simulink model "sampleModel1855"  (R2023a)
settings: Solver=VariableStepAuto  StartTime=0.0  StopTime=10.0  RelTol=1e-3
libraries: hdlsllib x4, simulink x1
settings Model: Creator=user1  LastModifiedBy=user1

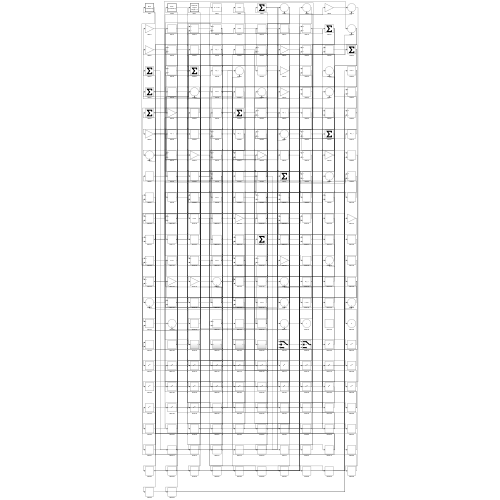
[thumbnail: Simulink's stored preview of the top-level diagram]
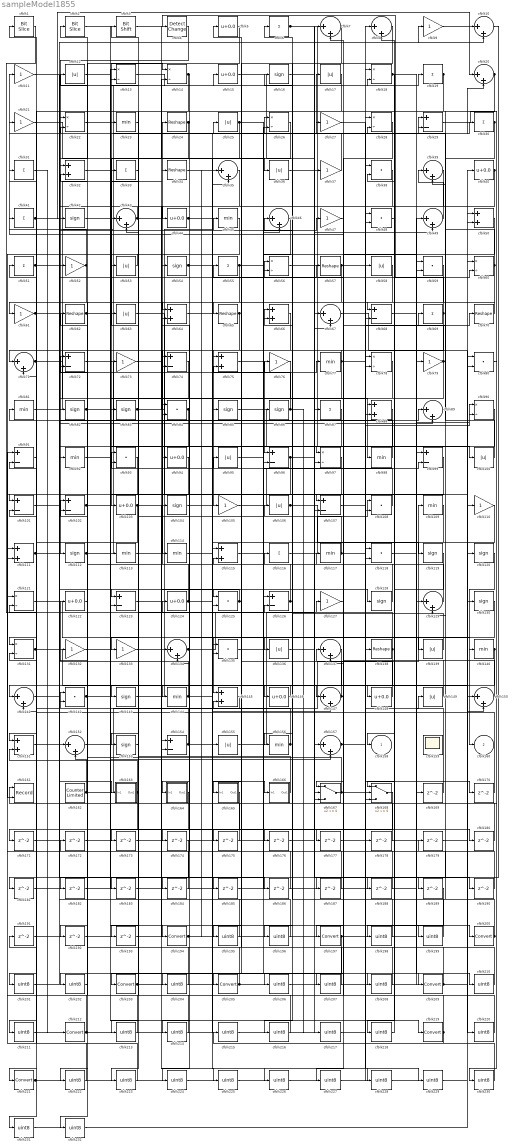
== system sampleModel1855 ==
  cfblk1 : hdlsllib/Logic and Bit Operations/Bit Slice  lidx=7  ridx=0
  cfblk{7..8,10,20,35,39,43,46,49,67,71,89,129,134,137,141,147,150,152,157} (20 alike) : Sum  Inputs=|++
  cfblk{12,17,25,36,53,58,63,95,100,106,136,139,149,155} (14 alike) : Abs  SaturateOnIntegerOverflow=off
  cfblk{29,68,72,74,91,96,99,101..102,107,123,126,154} (13 alike) : Sum  Inputs=+-
  cfblk{5,15,40,44,94,103,122,124,146,148} (10 alike) : Bias  Bias=0.0  SaturateOnIntegerOverflow=off
  cfblk{16,42,54,82..83,85..86,104,112,119..120,128,130,143,153} (15 alike) : Signum
  cfblk{9,11,21,27,37,47,52,61,73,76,79,105,110,127,132..133} (16 alike) : Gain
  cfblk{38,48,59,80,84,93,108,118,125,135,142} (11 alike) : DotProduct  OutDataTypeStr=Inherit: Inherit via internal rule
  cfblk{23,45,77,81,92,98,109,113..114,117,140,144,156} (13 alike) : MinMax
  cfblk{32,50,64,66,75,88,111,115,145,151} (10 alike) : Sum
  cfblk{6,19,30..31,33,41,51,55,69,87,116} (11 alike) : Sum  Inputs=+
  cfblk{13..14,18,22,26,28,56,60,78,90,97,121,131} (13 alike) : Product  Inputs=*/  RndMeth=Zero  SaturateOnIntegerOverflow=on
  cfblk{24,34,57,62,65,70,138} (7 alike) : Reshape
  cfblk159 : Scope
      settings: Floating=on
  cfblk161 : Record  FileSettingsInternal="{\"entries\":[{\"content\":{\"excelSettings\":{\"content\":{},\"type\":\"Streamout.ExcelSettings\"}},\"type\":\"Streamout.FileSettingStorage\",\"uuid\":\"\"}],\"packageUris\":[\"http:\\/\\/schema.mathworks.com\\/mf0\\/streamout_blocks\\/R2020a\"],\"version\":\"1.0\"}"  Layout=[1 1]  SignalsInternal="{\"entries\":[{\"content\":{\"signals\":[{\"content\":{\"blockPath\":[],\"dimensions\":[1],\"domain\":\"\",\"lineColor\":\"#a2142f\",\"plots\":[1],\"port\":1,\"signalID\":4583,\"signalName\":\"XY Graph:1\"},\"type\":\"RecordBlkView.Signal\",\"uuid\":\"\"},{\"content\":{\"blockPath\":[],\"dimensions\":[1],\"domain\":\"\",\"lineColor\":\"#139fff\",\"plots\":[1],\"port\":2,\"signalID\":4586,\"signalName\":\"XY Graph:2\"},\"type\":\"RecordBlkView.Signal\",\"uuid\":\"\"}]},\"type\":\"RecordBlkView.InputSignals\",\"uuid\":\"\"}],\"packageUris\":[\"http:\\/\\/schema.mathworks.com\\/mf0\\/streamout_blocks\\/R2020a\"],\"version\":\"1.0\"}"  VisualizationBindings="{\"xyplotplugin\":{\"info\":[{\"series\":[{\"bindingParametersList\":[{\"parameter\":\"X-Axis\",\"signalID\":4583,\"signalName\":\"XY Graph:1\"},{\"parameter\":\"Y-Axis\",\"signalID\":4586,\"signalName\":\"XY Graph:2\"}],\"seriesID\":3275}],\"subplotID\":1}]}}"  CompatibilityTag=XY  st=-1
  cfblk162 : hdlsllib/Sources/Counter Limited  uplimit=7  tsamp=-1
  cfblk163 : Subsystem
      settings: LibrarySourceBlock=|
      | hdlsllib/Ports &
      | Subsystems/Subsystem
  cfblk164 : Subsystem
      settings: LibrarySourceBlock=|
      | hdlsllib/Ports &
      | Subsystems/Subsystem
  cfblk165 : Subsystem
      settings: LibrarySourceBlock=|
      | hdlsllib/Ports &
      | Subsystems/Subsystem
  cfblk166 : Subsystem
      settings: LibrarySourceBlock=|
      | hdlsllib/Ports &
      | Subsystems/Subsystem
  cfblk167 : Switch  SaturateOnIntegerOverflow=off  InputSameDT=off
  cfblk168 : Switch  SaturateOnIntegerOverflow=off  InputSameDT=off
  cfblk{169..193} (25 alike) : Delay  SampleTime=1
  cfblk{194,197,200,203,205,209,212,219,221} (9 alike) : DataTypeConversion  SaturateOnIntegerOverflow=off  RndMeth=Floor
  cfblk{195..196,198..199,201..202,204,206..208,210..211,213..218,220,222..232} (30 alike) : DataTypeConversion  OutDataTypeStr=uint8  SaturateOnIntegerOverflow=off  RndMeth=Floor
  cfblk2 : hdlsllib/Logic and Bit Operations/Bit Slice  lidx=7  ridx=0
  cfblk3 : hdlsllib/Logic and Bit Operations/Bit Shift  mode=Shift Left Logical  N=0
  cfblk4 : simulink/Logic and Bit Operations/Detect Change  vinit=0  OutDataTypeStr=boolean
      settings: LibrarySourceBlock=|
      | hdlsllib/Logic and Bit
      | Operations/Detect
      | Change
  cfblk158 : Outport  VectorParamsAs1DForOutWhenUnconnected=off
  cfblk160 : Outport  Port=2  VectorParamsAs1DForOutWhenUnconnected=off
  wires:
  cfblk86/1 -> cfblk75/2, cfblk217/1
  cfblk65/1 -> cfblk105/1, cfblk74/2
  cfblk112/1 -> cfblk15/1, cfblk54/1
  cfblk48/1 -> cfblk97/1
  cfblk126/1 -> cfblk24/1, cfblk106/1
  cfblk62/1 -> cfblk14/1, cfblk2/1
  cfblk26/1 -> cfblk103/1
  cfblk69/1 -> cfblk4/1, cfblk151/1, cfblk187/1
  cfblk4/1 -> cfblk112/1
  cfblk28/1 -> cfblk197/1
  cfblk120/1 -> cfblk160/1
  cfblk125/1 -> cfblk123/1, cfblk185/1
  cfblk19/1 -> cfblk71/1, cfblk211/1, cfblk218/1
  cfblk71/1 -> cfblk34/1, cfblk57/1
  cfblk143/1 -> cfblk45/1
  cfblk156/1 -> cfblk142/1, cfblk51/1
  cfblk43/1 -> cfblk42/1, cfblk176/1
  cfblk84/1 -> cfblk92/1, cfblk102/2
  cfblk72/1 -> cfblk97/2
  cfblk148/1 -> cfblk137/1
  cfblk116/1 -> cfblk108/1
  cfblk30/1 -> cfblk145/1, cfblk189/1
  cfblk74/1 -> cfblk83/1
  cfblk1/1 -> cfblk124/1
  cfblk146/1 -> cfblk143/1
  cfblk88/1 -> cfblk165/1(In1)
  cfblk167/1 -> cfblk12/1, cfblk149/1
  cfblk22/1 -> cfblk194/1
  cfblk66/1 -> cfblk114/1
  cfblk52/1 -> cfblk11/1, cfblk71/2
  cfblk12/1 -> cfblk113/1
  cfblk123/1 -> cfblk148/1
  cfblk25/1 -> cfblk59/2, cfblk204/1
  cfblk58/1 -> cfblk108/2
  cfblk29/1 -> cfblk161/1
  cfblk75/1 -> cfblk96/1
  cfblk81/1 -> cfblk30/1
  cfblk121/1 -> cfblk140/1
  cfblk145/1 -> cfblk142/2
  cfblk41/1 -> cfblk20/1, cfblk88/1
  cfblk5/1 -> cfblk32/1
  cfblk47/1 -> cfblk167/1
  cfblk149/1 -> cfblk55/1
  cfblk141/1 -> cfblk53/1
  cfblk93/1 -> cfblk101/1
  cfblk153/1 -> cfblk3/1
  cfblk40/1 -> cfblk44/1, cfblk75/1
  cfblk133/1 -> cfblk104/1
  cfblk46/1 -> cfblk96/2
  cfblk7/1 -> cfblk195/1, cfblk206/1
  cfblk55/1 -> cfblk82/1, cfblk46/2
  cfblk24/1 -> cfblk133/1, cfblk64/1
  cfblk54/1 -> cfblk128/1, cfblk35/2
  cfblk6/1 -> cfblk100/1, cfblk49/2
  cfblk64/1 -> cfblk155/1
  cfblk155/1 -> cfblk37/1
  cfblk61/1 -> cfblk118/1, cfblk163/1(In1), cfblk10/2
  cfblk142/1 -> cfblk126/2, cfblk84/2
  cfblk63/1 -> cfblk120/1
  cfblk117/1 -> cfblk66/1, cfblk33/1, cfblk70/1
  cfblk57/1 -> cfblk61/1, cfblk9/1
  cfblk23/1 -> cfblk203/1
  cfblk82/1 -> cfblk94/1, cfblk192/1, cfblk222/1
  cfblk139/1 -> cfblk46/1
  cfblk13/1 -> cfblk19/1
  cfblk163/1(Out1) -> cfblk151/2, cfblk201/1
  cfblk97/1 -> cfblk136/1
  cfblk44/1 -> cfblk146/1, cfblk88/2, cfblk199/1
  cfblk32/1 -> cfblk20/2
  cfblk102/1 -> cfblk107/1, cfblk72/1
  cfblk37/1 -> cfblk5/1
  cfblk135/1 -> cfblk209/1
  cfblk140/1 -> cfblk158/1, cfblk171/1
  cfblk3/1 -> cfblk36/1
  cfblk56/1 -> cfblk60/2
  cfblk51/1 -> cfblk17/1, cfblk18/2
  cfblk49/1 -> cfblk39/1
  cfblk103/1 -> cfblk125/1, cfblk231/1
  cfblk70/1 -> cfblk65/1
  cfblk144/1 -> cfblk122/1, cfblk63/1, cfblk76/1
  cfblk111/1 -> cfblk47/1, cfblk123/2
  cfblk162/1 -> cfblk109/1, cfblk131/2
  cfblk128/1 -> cfblk116/1
  cfblk130/1 -> cfblk164/1(In1)
  cfblk132/1 -> cfblk219/1
  cfblk106/1 -> cfblk119/1, cfblk66/2
  cfblk99/1 -> cfblk111/2
  cfblk151/1 -> cfblk89/1
  cfblk21/1 -> cfblk115/1
  cfblk53/1 -> cfblk52/1
  cfblk20/1 -> cfblk68/1, cfblk129/2
  cfblk129/1 -> cfblk6/1
  cfblk137/1 -> cfblk141/1
  cfblk134/1 -> cfblk139/1, cfblk86/1
  cfblk115/1 -> cfblk99/2
  cfblk94/1 -> cfblk141/2
  cfblk108/1 -> cfblk93/1
  cfblk17/1 -> cfblk84/1
  cfblk36/1 -> cfblk157/1
  cfblk9/1 -> cfblk10/1
  cfblk152/1 -> cfblk200/1
  cfblk91/1 -> cfblk221/1
  cfblk124/1 -> cfblk56/1, cfblk72/2
  cfblk15/1 -> cfblk67/2
  cfblk85/1 -> cfblk130/1
  cfblk98/1 -> cfblk81/1
  cfblk18/1 -> cfblk168/1, cfblk210/1
  cfblk114/1 -> cfblk26/1
  cfblk136/1 -> cfblk29/1
  cfblk77/1 -> cfblk74/1, cfblk144/1, cfblk229/1
  cfblk96/1 -> cfblk131/1, cfblk190/1
  cfblk157/1 -> cfblk117/1, cfblk90/2
  cfblk33/1 -> cfblk73/1
  cfblk67/1 -> cfblk150/2
  cfblk154/1 -> cfblk93/2, cfblk166/1(In1)
  cfblk147/1 -> cfblk95/1, cfblk27/1
  cfblk38/1 -> cfblk68/2
  cfblk14/1 -> cfblk173/1, cfblk174/1
  cfblk45/1 -> cfblk161/2
  cfblk131/1 -> cfblk89/2, cfblk220/1
  cfblk90/1 -> cfblk147/1
  cfblk166/1(Out1) -> cfblk43/2
  cfblk105/1 -> cfblk18/1
  cfblk109/1 -> cfblk125/2
  cfblk100/1 -> cfblk69/1
  cfblk118/1 -> cfblk90/1
  cfblk83/1 -> cfblk14/2, cfblk138/1
  cfblk150/1 -> cfblk7/2
  cfblk110/1 -> cfblk205/1
  cfblk89/1 -> cfblk29/2
  cfblk35/1 -> cfblk154/2
  cfblk79/1 -> cfblk39/2, cfblk98/1, cfblk41/1, cfblk134/2
  cfblk122/1 -> cfblk102/1
  cfblk101/1 -> cfblk77/1
  cfblk92/1 -> cfblk157/2
  cfblk31/1 -> cfblk212/1
  cfblk76/1 -> cfblk153/1
  cfblk60/1 -> cfblk21/1, cfblk156/1
  cfblk34/1 -> cfblk147/2
  cfblk138/1 -> cfblk13/2, cfblk168/3
  cfblk68/1 -> cfblk169/1
  cfblk169/1 -> cfblk99/1
  cfblk107/1 -> cfblk170/1
  cfblk170/1 -> cfblk1/1
  cfblk171/1 -> cfblk167/2
  cfblk172/1 -> cfblk56/2
  cfblk173/1 -> cfblk7/1
  cfblk42/1 -> cfblk175/1
  cfblk175/1 -> cfblk101/2
  cfblk95/1 -> cfblk177/1
  cfblk177/1 -> cfblk60/1
  cfblk27/1 -> cfblk178/1
  cfblk178/1 -> cfblk145/2
  cfblk179/1 -> cfblk150/1
  cfblk16/1 -> cfblk180/1
  cfblk180/1 -> cfblk154/1
  cfblk10/1 -> cfblk181/1
  cfblk181/1 -> cfblk13/1
  cfblk59/1 -> cfblk182/1
  cfblk182/1 -> cfblk129/1
  cfblk168/1 -> cfblk183/1
  cfblk183/1 -> cfblk67/1
  cfblk11/1 -> cfblk184/1
  cfblk184/1 -> cfblk111/1
  cfblk185/1 -> cfblk26/2
  cfblk73/1 -> cfblk186/1
  cfblk186/1 -> cfblk32/2
  cfblk187/1 -> cfblk64/2
  cfblk119/1 -> cfblk188/1
  cfblk188/1 -> cfblk126/1
  cfblk190/1 -> cfblk115/2
  cfblk191/1 -> cfblk134/1
  cfblk192/1 -> cfblk167/3
  cfblk164/1(Out1) -> cfblk193/1
  cfblk193/1 -> cfblk85/1
  cfblk194/1 -> cfblk118/2, cfblk35/1
  cfblk195/1 -> cfblk22/1
  cfblk176/1 -> cfblk196/1
  cfblk196/1 -> cfblk22/2
  cfblk197/1 -> cfblk79/1, cfblk232/1
  cfblk189/1 -> cfblk198/1
  cfblk198/1 -> cfblk28/1
  cfblk199/1 -> cfblk28/2
  cfblk200/1 -> cfblk179/1, cfblk16/1
  cfblk201/1 -> cfblk152/1
  cfblk165/1(Out1) -> cfblk202/1
  cfblk202/1 -> cfblk152/2
  cfblk203/1 -> cfblk58/1, cfblk226/1
  cfblk204/1 -> cfblk23/1
  cfblk205/1 -> cfblk172/1, cfblk49/1
  cfblk206/1 -> cfblk110/1
  cfblk127/1 -> cfblk207/1
  cfblk207/1 -> cfblk25/1
  cfblk2/1 -> cfblk208/1
  cfblk208/1 -> cfblk127/1
  cfblk209/1 -> cfblk59/1, cfblk38/2
  cfblk210/1 -> cfblk135/1
  cfblk211/1 -> cfblk135/2
  cfblk212/1 -> cfblk121/2, cfblk107/2
  cfblk39/1 -> cfblk213/1
  cfblk213/1 -> cfblk31/1
  cfblk87/1 -> cfblk214/1
  cfblk214/1 -> cfblk62/1
  cfblk215/1 -> cfblk87/1
  cfblk8/1 -> cfblk216/1
  cfblk216/1 -> cfblk43/1
  cfblk217/1 -> cfblk8/1
  cfblk218/1 -> cfblk8/2
  cfblk219/1 -> cfblk215/1, cfblk191/1, cfblk137/2, cfblk121/1
  cfblk220/1 -> cfblk132/1
  cfblk221/1 -> cfblk168/2, cfblk40/1
  cfblk222/1 -> cfblk91/1
  cfblk174/1 -> cfblk223/1
  cfblk223/1 -> cfblk91/2
  cfblk78/1 -> cfblk224/1
  cfblk224/1 -> cfblk38/1
  cfblk113/1 -> cfblk225/1
  cfblk225/1 -> cfblk78/1
  cfblk226/1 -> cfblk78/2
  cfblk50/1 -> cfblk227/1
  cfblk227/1 -> cfblk48/2
  cfblk104/1 -> cfblk228/1
  cfblk228/1 -> cfblk50/1
  cfblk229/1 -> cfblk50/2
  cfblk80/1 -> cfblk230/1
  cfblk230/1 -> cfblk48/1
  cfblk231/1 -> cfblk80/1
  cfblk232/1 -> cfblk80/2

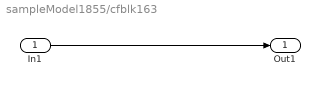
== system sampleModel1855/cfblk163 ==
  In1 : Inport
  Out1 : Outport
  wires:
  In1/1 -> Out1/1

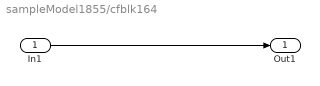
== system sampleModel1855/cfblk164 ==
  In1 : Inport
  Out1 : Outport
  wires:
  In1/1 -> Out1/1

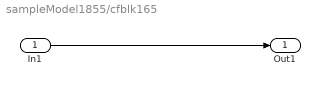
== system sampleModel1855/cfblk165 ==
  In1 : Inport
  Out1 : Outport
  wires:
  In1/1 -> Out1/1

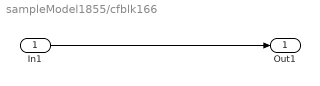
== system sampleModel1855/cfblk166 ==
  In1 : Inport
  Out1 : Outport
  wires:
  In1/1 -> Out1/1
